simulink model "Inertial_Compensation_Test1"  (R2020a)
settings: Solver=VariableStepAuto  StartTime=0.0  StopTime=20.0  RelTol=1e-3
libraries: dsparch4 x7
settings Model: Creator=bread  LastModifiedBy=bread

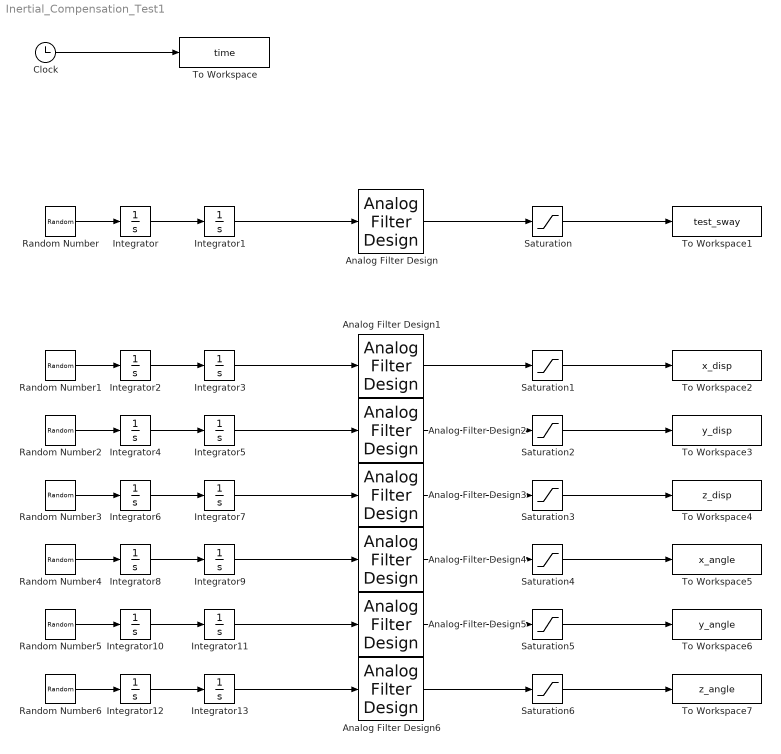
== system Inertial_Compensation_Test1 ==
  Analog Filter Design{,1..6} (7 alike) : dsparch4/Analog Filter Design  method=Butterworth  filttype=Highpass  N=2  Wlo=1.319468913  Whi=80  Rp=2  Rs=40
  Clock : Clock
  Integrator{,1..13} (14 alike) : Integrator
  Random Number : RandomNumber  Variance=0.5  Seed=1  SampleTime=0.0033
  Random Number1 : RandomNumber  Variance=12  Seed=107  SampleTime=0.0033
  Random Number2 : RandomNumber  Variance=9  Seed=108  SampleTime=0.0033
  Random Number3 : RandomNumber  Variance=12  Seed=109  SampleTime=0.0033
  Random Number4 : RandomNumber  Variance=60000  Seed=110  SampleTime=0.0033
  Random Number5 : RandomNumber  Variance=70000  Seed=111  SampleTime=0.0033
  Random Number6 : RandomNumber  Variance=60000  Seed=112  SampleTime=0.0033
  Saturation : Saturate  UpperLimit=0.05  LowerLimit=-0.05
  Saturation1 : Saturate  UpperLimit=0.22  LowerLimit=-0.22
  Saturation2 : Saturate  UpperLimit=0.2  LowerLimit=-0.18
  Saturation3 : Saturate  UpperLimit=0.22  LowerLimit=-0.27
  Saturation4 : Saturate  UpperLimit=17  LowerLimit=-17
  Saturation5 : Saturate  UpperLimit=19  LowerLimit=-19
  Saturation6 : Saturate  UpperLimit=17  LowerLimit=-17
  To Workspace : ToWorkspace  VariableName=time  SaveFormat=Timeseries  SampleTime=-1
  To Workspace1 : ToWorkspace  VariableName=test_sway  SaveFormat=Timeseries  SampleTime=-1
  To Workspace2 : ToWorkspace  VariableName=x_disp  SaveFormat=Timeseries  SampleTime=-1
  To Workspace3 : ToWorkspace  VariableName=y_disp  SaveFormat=Timeseries  SampleTime=-1
  To Workspace4 : ToWorkspace  VariableName=z_disp  SaveFormat=Timeseries  SampleTime=-1
  To Workspace5 : ToWorkspace  VariableName=x_angle  SaveFormat=Timeseries  SampleTime=-1
  To Workspace6 : ToWorkspace  VariableName=y_angle  SaveFormat=Timeseries  SampleTime=-1
  To Workspace7 : ToWorkspace  VariableName=z_angle  SaveFormat=Timeseries  SampleTime=-1
  wires:
  Clock/1 -> To Workspace/1
  Random Number/1 -> Integrator/1
  Integrator/1 -> Integrator1/1
  Integrator1/1 -> Analog Filter Design/1
  Analog Filter Design/1 -> Saturation/1
  Saturation/1 -> To Workspace1/1
  Analog Filter Design1/1 -> Saturation1/1
  Integrator3/1 -> Analog Filter Design1/1
  Integrator2/1 -> Integrator3/1
  Saturation1/1 -> To Workspace2/1
  Random Number1/1 -> Integrator2/1
  Analog Filter Design2/1 -> Saturation2/1
  Integrator5/1 -> Analog Filter Design2/1
  Integrator4/1 -> Integrator5/1
  Saturation2/1 -> To Workspace3/1
  Random Number2/1 -> Integrator4/1
  Analog Filter Design3/1 -> Saturation3/1
  Integrator7/1 -> Analog Filter Design3/1
  Integrator6/1 -> Integrator7/1
  Saturation3/1 -> To Workspace4/1
  Random Number3/1 -> Integrator6/1
  Analog Filter Design4/1 -> Saturation4/1
  Integrator9/1 -> Analog Filter Design4/1
  Integrator8/1 -> Integrator9/1
  Saturation4/1 -> To Workspace5/1
  Random Number4/1 -> Integrator8/1
  Analog Filter Design5/1 -> Saturation5/1
  Integrator11/1 -> Analog Filter Design5/1
  Integrator10/1 -> Integrator11/1
  Saturation5/1 -> To Workspace6/1
  Random Number5/1 -> Integrator10/1
  Analog Filter Design6/1 -> Saturation6/1
  Integrator13/1 -> Analog Filter Design6/1
  Integrator12/1 -> Integrator13/1
  Saturation6/1 -> To Workspace7/1
  Random Number6/1 -> Integrator12/1
